simulink model "GridN2"  (R2021a)
settings: Solver=FixedStepAuto  StartTime=0  StopTime=0.2  FixedStep=0.2  RelTol=1e-3
libraries: spsDistributedParametersLineLib x32, spsThreePhaseSeriesRLCLoadLib x10, spsThreePhaseVIMeasurementLib x2, spsGroundLib x1, spsThreePhaseSourceLib x1, spsSeriesRLCBranchLib x1, spspowerguiLib x1
settings Model: Creator=miair  LastModifiedBy=Admin
settings SolverCC: AlgebraicLoopSolver=TrustRegion
settings DebuggingCC: SFMachineParentedDataDiag=warning  ArithmeticOperatorsInVariantConditions=warning
settings SFSimCC: SimUseLocalCustomCode=off  CustomCodeUndefinedFunction=UseInterfaceOnly
settings RTWCC: RTWUseLocalCustomCode=off
settings CodeAppCC: StateflowObjectComments=on
settings SimscapeCC: SimscapeNormalizeSystem=off

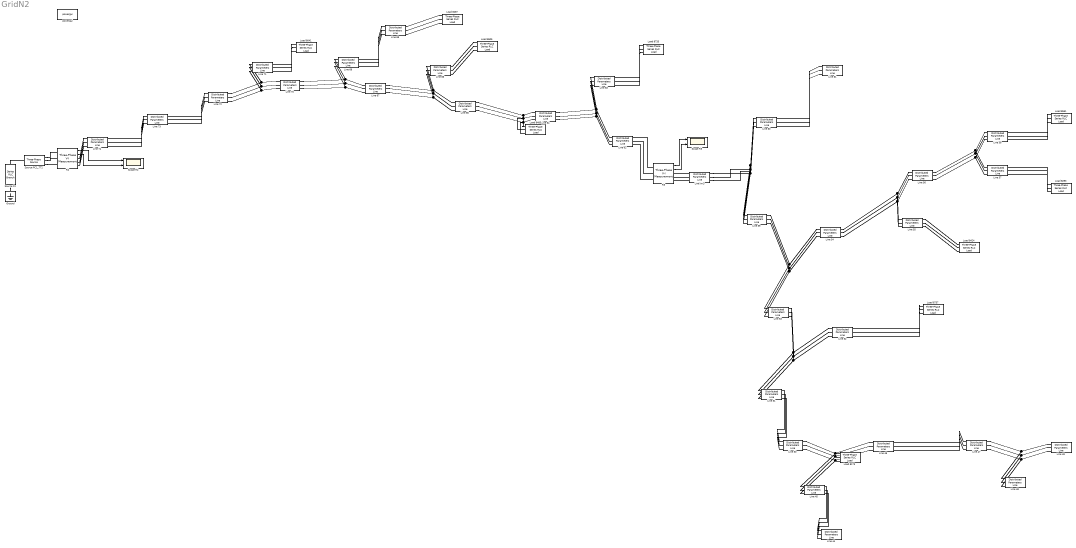
== system GridN2 ==
  Ground : spsGroundLib/Ground  LConnTagsString=a
  Line 44 : spsDistributedParametersLineLib/Distributed Parameters Line  Phases=3  Length=1.11  Frequency=50  Resistance=[0.502970710632245 0.0486237908083191 0.0486712220507153;0.0486237908083191 0.502875844822084 0.0486237934466192;0.0486712220507153 0.0486237934466192 0.502970710632245]  Inductance=[0.00286900545038753 0.00133270803418135 0.00132951476746136;0.00133270803418135 0.00286931445999602 0.00133799988507366;0.00132951476746136 0.00133799988507366 0.00286900545038753]  Capacitance=[8.11484299003193e-09 -1.94249816214699e-09 -1.86930692621136e-09;-1.94249816214699e-09 8.0425699231653e-09 -1.98049571960044e-09;-1.86930692621136e-09 -1.98049571960044e-09 8.13337738722527e-09]  x1=[235.499197131344 9974.6534173124 9973.62003670647;314.159265358979 314.159265358979 314.159265358979;0.999986971190447 -0.174358854278801 -1.7453327880671]  x2=[235.499532901852 9974.66274518172 9973.62938461404;314.159265358979 314.159265358979 314.159265358979;0.999986478978544 -0.1743597320809 -1.74533367343035]  x3=[0.20646047330324 25.3733648317573 25.5655395365313;314.159265358979 314.159265358979 314.159265358979;0.998298068545493 -0.17572688726887 -1.74670236391409]  x4=[0.206460473415381 25.3733648393287 25.5655395441195;314.159265358979 314.159265358979 314.159265358979;0.999986479195967 -0.174359732083028 -1.74533367343085]  x5=5.37516004033389e-06  V1=ones(3,3)  V2=ones(3,3)  I1=ones(3,3)  I2=ones(3,3)  nHarmo=1  Measurements=None  Decoupling=off  VsMag0=0  VrMag0=0  VsAngle0=0  VrAngle0=0  IsMag0=0  IrMag0=0  IsAngle0=0  IrAngle0=0
      settings: SourceProductBaseCode=PS
  Line 45 : spsDistributedParametersLineLib/Distributed Parameters Line  Phases=3  Length=0.03  Frequency=50  Resistance=[0.476003738225748 0.351747138225748 0.351747138225748;0.351747138225748 0.476003738225748 0.351747138225748;0.351747138225748 0.351747138225748 0.476003738225748]  Inductance=[0.000705954362986426 0.000459934243504405 0.000459934243504405;0.000459934243504405 0.000705954362986426 0.000459934243504405;0.000459934243504405 0.000459934243504405 0.000705954362986426]  Capacitance=[5.7561313269996e-07 -1.37543883484145e-07 -1.37543912800485e-07;-1.37543883484145e-07 5.75613027339387e-07 -1.37543875208088e-07;-1.37543912800485e-07 -1.37543875208088e-07 5.75613005057695e-07]  x1=[0.394611268706457 9975.72744348311 9975.73788089302;314.159265358979 314.159265358979 314.159265358979;1.53603881552804 -0.0977008679647626 -1.66848911141861]  x2=[0.394608901343207 9975.72760187554 9975.73803973793;314.159265358979 314.159265358979 314.159265358979;1.53600998571819 -0.0977008934643248 -1.66848913704469]  x3=[0.00519543625612021 537.015102166399 537.015558234621;314.159265358979 314.159265358979 314.159265358979;1.48851023303865 -0.0978903869659834 -1.66867918632059]  x4=[0.0055420607596715 537.015037865136 537.015622619077;314.159265358979 314.159265358979 314.159265358979;1.58036294124239 -0.0976362193465509 -1.66842390704819]  x5=6.63129528657629e-07  V1=ones(3,3)  V2=ones(3,3)  I1=ones(3,3)  I2=ones(3,3)  nHarmo=1  Measurements=None  Decoupling=off  VsMag0=0  VrMag0=0  VsAngle0=0  VrAngle0=0  IsMag0=0  IrMag0=0  IsAngle0=0  IrAngle0=0
      settings: SourceProductBaseCode=PS
  Line 46 : spsDistributedParametersLineLib/Distributed Parameters Line  Phases=3  Length=0.28  Frequency=50  Resistance=[0.476003738225748 0.351747138225748 0.351747138225748;0.351747138225748 0.476003738225748 0.351747138225748;0.351747138225748 0.351747138225748 0.476003738225748]  Inductance=[0.000705954362986426 0.000459934243504405 0.000459934243504405;0.000459934243504405 0.000705954362986426 0.000459934243504405;0.000459934243504405 0.000459934243504405 0.000705954362986426]  Capacitance=[5.7561313269996e-07 -1.37543883484145e-07 -1.37543912800485e-07;-1.37543883484145e-07 5.75613027339387e-07 -1.37543875208088e-07;-1.37543912800485e-07 -1.37543875208088e-07 5.75613005057695e-07]  x1=[0.394611268706457 9975.72744348312 9975.73788089302;314.159265358979 314.159265358979 314.159265358979;1.5343027464817 -0.0987411899313736 -1.6695294333048]  x2=[0.394596540852003 9975.73476310246 9975.7452035338;314.159265358979 314.159265358979 314.159265358979;1.53410803074215 -0.0987423693851286 -1.66953061358232]  x3=[0.0052281315001106 536.342337149453 536.342813729589;314.159265358979 314.159265358979 314.159265358979;1.49901674095737 -0.0999540083208943 -1.67074264139569]  x4=[0.00547168054822011 536.342293969161 536.342857334771;314.159265358979 314.159265358979 314.159265358979;1.56592395108104 -0.0986952571936451 -1.66948311170117]  x5=6.18920893413787e-06  V1=ones(3,3)  V2=ones(3,3)  I1=ones(3,3)  I2=ones(3,3)  nHarmo=1  Measurements=None  Decoupling=off  VsMag0=0  VrMag0=0  VsAngle0=0  VrAngle0=0  IsMag0=0  IrMag0=0  IsAngle0=0  IrAngle0=0
      settings: SourceProductBaseCode=PS
  Line 47 : spsDistributedParametersLineLib/Distributed Parameters Line  Phases=3  Length=0.28  Frequency=50  Resistance=[0.646656091154803 0.0486237908083191 0.0486712220507153;0.0486237908083191 0.646561225344642 0.0486237934466192;0.0486712220507153 0.0486237934466192 0.646656091154803]  Inductance=[0.00282448912315926 0.00133270803418135 0.00132951476746136;0.00133270803418135 0.00282479813276775 0.00133799988507366;0.00132951476746136 0.00133799988507366 0.00282448912315926]  Capacitance=[7.89543174552926e-09 -1.85986777702161e-09 -1.7901190036642e-09;-1.85986777702161e-09 7.82540023894543e-09 -1.8957321828871e-09;-1.7901190036642e-09 -1.8957321828871e-09 7.91264394645417e-09]  x1=[130.165270523337 9974.69985442641 9973.79793227893;314.159265358979 314.159265358979 314.159265358979;1.01815520413661 -0.17955738670952 -1.75050430629446]  x2=[130.1653269492 9974.70262298928 9973.80070570772;314.159265358979 314.159265358979 314.159265358979;1.01815501889747 -0.179557739858097 -1.75050466239578]  x3=[0.113793008832073 25.3764192511602 25.5689515866396;314.159265358979 314.159265358979 314.159265358979;1.01691737955787 -0.180553856209588 -1.75150165648101]  x4=[0.113792232457286 25.3764196987183 25.5689511658165;314.159265358979 314.159265358979 314.159265358979;1.01897135143641 -0.178896144175293 -1.74984250504318]  x5=1.34161235953112e-06  V1=ones(3,3)  V2=ones(3,3)  I1=ones(3,3)  I2=ones(3,3)  nHarmo=1  Measurements=None  Decoupling=off  VsMag0=0  VrMag0=0  VsAngle0=0  VrAngle0=0  IsMag0=0  IrMag0=0  IsAngle0=0  IrAngle0=0
      settings: SourceProductBaseCode=PS
  Line 48 : spsDistributedParametersLineLib/Distributed Parameters Line  Phases=3  Length=0.3  Frequency=50  Resistance=[0.80718830189013 0.0486237908083191 0.0486712220507153;0.0486237908083191 0.807093436079969 0.0486237934466192;0.0486712220507153 0.0486237934466192 0.80718830189013]  Inductance=[0.00279786707424938 0.00133270803418135 0.00132951476746136;0.00133270803418135 0.00279817608385787 0.00133799988507366;0.00132951476746136 0.00133799988507366 0.00279786707424938]  Capacitance=[7.73340098830622e-09 -1.79942827973291e-09 -1.73218055098733e-09;-1.79942827973291e-09 7.66505189233746e-09 -1.83375898618858e-09;-1.73218055098733e-09 -1.83375898618858e-09 7.749673531177e-09]  x1=[52.3203507574151 9974.78925458762 9973.95475226715;314.159265358979 314.159265358979 314.159265358979;1.07773858299054 -0.18388639186805 -1.75479371977811]  x2=[52.3203560131605 9974.78987075889 9973.95536942842;314.159265358979 314.159265358979 314.159265358979;1.07773853006996 -0.183886493366591 -1.75479382212189]  x3=[0.0455873088828184 25.3094904148269 25.5001937895356;314.159265358979 314.159265358979 314.159265358979;1.0772903311148 -0.18423793333454 -1.75514555863699]  x4=[0.0455873088210403 25.3094904150667 25.5001937897322;314.159265358979 314.159265358979 314.159265358979;1.0777385304448 -0.183886493366644 -1.75479382212035]  x5=1.42674452918375e-06  V1=ones(3,3)  V2=ones(3,3)  I1=ones(3,3)  I2=ones(3,3)  nHarmo=1  Measurements=None  Decoupling=off  VsMag0=0  VrMag0=0  VsAngle0=0  VrAngle0=0  IsMag0=0  IrMag0=0  IsAngle0=0  IrAngle0=0
      settings: SourceProductBaseCode=PS
  Line 49 : spsDistributedParametersLineLib/Distributed Parameters Line  Phases=3  Length=0.26  Frequency=50  Resistance=[0.646656091154803 0.0486237908083191 0.0486712220507153;0.0486237908083191 0.646561225344642 0.0486237934466192;0.0486712220507153 0.0486237934466192 0.646656091154803]  Inductance=[0.00282448912315926 0.00133270803418135 0.00132951476746136;0.00133270803418135 0.00282479813276775 0.00133799988507366;0.00132951476746136 0.00133799988507366 0.00282448912315926]  Capacitance=[7.89543174552926e-09 -1.85986777702161e-09 -1.7901190036642e-09;-1.85986777702161e-09 7.82540023894543e-09 -1.8957321828871e-09;-1.7901190036642e-09 -1.8957321828871e-09 7.91264394645417e-09]  x1=[130.165326949199 9974.70262298928 9973.80070570772;314.159265358979 314.159265358979 314.159265358979;1.01818512460841 -0.179533822848032 -1.75048072261842]  x2=[130.16533691815 9974.70310512625 9973.80118871937;314.159265358979 314.159265358979 314.159265358979;1.01818509158021 -0.179533884346449 -1.75048078463717]  x3=[0.113793699489359 25.3769942885345 25.569534921312;314.159265358979 314.159265358979 314.159265358979;1.0177937339126 -0.179844774725389 -1.75079197073384]  x4=[0.113793699536148 25.3769942886748 25.569534921511;314.159265358979 314.159265358979 314.159265358979;1.01818509150153 -0.179533884349861 -1.75048078463657]  x5=1.2457829052789e-06  V1=ones(3,3)  V2=ones(3,3)  I1=ones(3,3)  I2=ones(3,3)  nHarmo=1  Measurements=None  Decoupling=off  VsMag0=0  VrMag0=0  VsAngle0=0  VrAngle0=0  IsMag0=0  IrMag0=0  IsAngle0=0  IrAngle0=0
      settings: SourceProductBaseCode=PS
  Line 50 : spsDistributedParametersLineLib/Distributed Parameters Line  Phases=3  Length=0.02  Frequency=50  Resistance=[0.476003738225748 0.351747138225748 0.351747138225748;0.351747138225748 0.476003738225748 0.351747138225748;0.351747138225748 0.351747138225748 0.476003738225748]  Inductance=[0.000705954362986426 0.000459934243504405 0.000459934243504405;0.000459934243504405 0.000705954362986426 0.000459934243504405;0.000459934243504405 0.000459934243504405 0.000705954362986426]  Capacitance=[5.7561313269996e-07 -1.37543883484145e-07 -1.37543912800485e-07;-1.37543883484145e-07 5.75613027339387e-07 -1.37543875208088e-07;-1.37543912800485e-07 -1.37543875208088e-07 5.75613005057695e-07]  x1=[0.394613836475679 9975.73127591054 9975.74171280773;314.159265358979 314.159265358979 314.159265358979;1.53614175066651 -0.0976590526065954 -1.66844729592049]  x2=[0.394611268706457 9975.72744348312 9975.73788089302;314.159265358979 314.159265358979 314.159265358979;1.5361082582899 -0.0976592550860982 -1.66844749854316]  x3=[0.00508627848822846 535.56585629888 535.566267206896;314.159265358979 314.159265358979 314.159265358979;1.45102711429053 -0.0975036292293395 -1.66829282028614]  x4=[0.00567610136422067 538.518382585317 538.519012218396;314.159265358979 314.159265358979 314.159265358979;1.61223031069708 -0.0978968261558066 -1.66868412697944]  x5=4.42086352438419e-07  V1=ones(3,3)  V2=ones(3,3)  I1=ones(3,3)  I2=ones(3,3)  nHarmo=1  Measurements=None  Decoupling=off  VsMag0=0  VrMag0=0  VsAngle0=0  VrAngle0=0  IsMag0=0  IrMag0=0  IsAngle0=0  IrAngle0=0
      settings: SourceProductBaseCode=PS
  Line 51 : spsDistributedParametersLineLib/Distributed Parameters Line  Phases=3  Length=1.71  Frequency=50  Resistance=[0.646656091154803 0.0486237908083191 0.0486712220507153;0.0486237908083191 0.646561225344642 0.0486237934466192;0.0486712220507153 0.0486237934466192 0.646656091154803]  Inductance=[0.00282448912315926 0.00133270803418135 0.00132951476746136;0.00133270803418135 0.00282479813276775 0.00133799988507366;0.00132951476746136 0.00133799988507366 0.00282448912315926]  Capacitance=[7.89543174552926e-09 -1.85986777702161e-09 -1.7901190036642e-09;-1.85986777702161e-09 7.82540023894543e-09 -1.8957321828871e-09;-1.7901190036642e-09 -1.8957321828871e-09 7.91264394645417e-09]  x1=[130.153869834393 9976.25230830841 9975.34909810887;314.159265358979 314.159265358979 314.159265358979;1.01593395982582 -0.181153028787364 -1.75210222449929]  x2=[130.165195828942 9974.6963681945 9973.79444148245;314.159265358979 314.159265358979 314.159265358979;1.01600469152128 -0.181266070959912 -1.75221461748997]  x3=[0.117758466924286 23.8642665109004 24.0560073748523;314.159265358979 314.159265358979 314.159265358979;0.996810443572246 -0.17982504524178 -1.7508416785956]  x4=[0.109697369932617 26.8098980337402 27.0019891541792;314.159265358979 314.159265358979 314.159265358979;1.03386689924875 -0.184375752260112 -1.75526795592347]  x5=8.19341833856506e-06  V1=ones(3,3)  V2=ones(3,3)  I1=ones(3,3)  I2=ones(3,3)  nHarmo=1  Measurements=None  Decoupling=off  VsMag0=0  VrMag0=0  VsAngle0=0  VrAngle0=0  IsMag0=0  IrMag0=0  IsAngle0=0  IrAngle0=0
      settings: SourceProductBaseCode=PS
  Line 52 : spsDistributedParametersLineLib/Distributed Parameters Line  Phases=3  Length=0.02  Frequency=50  Resistance=[0.646656091154803 0.0486237908083191 0.0486712220507153;0.0486237908083191 0.646561225344642 0.0486237934466192;0.0486712220507153 0.0486237934466192 0.646656091154803]  Inductance=[0.00282448912315926 0.00133270803418135 0.00132951476746136;0.00133270803418135 0.00282479813276775 0.00133799988507366;0.00132951476746136 0.00133799988507366 0.00282448912315926]  Capacitance=[7.89543174552926e-09 -1.85986777702161e-09 -1.7901190036642e-09;-1.85986777702161e-09 7.82540023894543e-09 -1.8957321828871e-09;-1.7901190036642e-09 -1.8957321828871e-09 7.91264394645417e-09]  x1=[130.153869834393 9976.25230830841 9975.34909810887;314.159265358979 314.159265358979 314.159265358979;1.0184778924009 -0.179132041436896 -1.75007931331198]  x2=[130.154016631798 9976.23079318743 9975.32762879486;314.159265358979 314.159265358979 314.159265358979;1.01847831718231 -0.179132357584775 -1.75007962248494]  x3=[0.116739942644273 24.1579696741118 24.3502140022841;314.159265358979 314.159265358979 314.159265358979;0.992668885557271 -0.149703484817279 -1.72089466112461]  x4=[0.110933827863639 26.6377132487628 26.8306479377076;314.159265358979 314.159265358979 314.159265358979;1.04560756980061 -0.205843471298248 -1.77658837325643]  x5=9.5829454252223e-08  V1=ones(3,3)  V2=ones(3,3)  I1=ones(3,3)  I2=ones(3,3)  nHarmo=1  Measurements=None  Decoupling=off  VsMag0=0  VrMag0=0  VsAngle0=0  VrAngle0=0  IsMag0=0  IrMag0=0  IsAngle0=0  IrAngle0=0
      settings: SourceProductBaseCode=PS
  Line 53 : spsDistributedParametersLineLib/Distributed Parameters Line  Phases=3  Length=0.02  Frequency=50  Resistance=[0.646656091154803 0.0486237908083191 0.0486712220507153;0.0486237908083191 0.646561225344642 0.0486237934466192;0.0486712220507153 0.0486237934466192 0.646656091154803]  Inductance=[0.00282448912315926 0.00133270803418135 0.00132951476746136;0.00133270803418135 0.00282479813276775 0.00133799988507366;0.00132951476746136 0.00133799988507366 0.00282448912315926]  Capacitance=[7.89543174552926e-09 -1.85986777702161e-09 -1.7901190036642e-09;-1.85986777702161e-09 7.82540023894543e-09 -1.8957321828871e-09;-1.7901190036642e-09 -1.8957321828871e-09 7.91264394645417e-09]  x1=[130.153585411917 9976.29177268076 9975.38850120097;314.159265358979 314.159265358979 314.159265358979;1.01847665737296 -0.179130371531821 -1.75007765770378]  x2=[130.153869834393 9976.25230830841 9975.34909810887;314.159265358979 314.159265358979 314.159265358979;1.0184778924009 -0.179132041436896 -1.75007931331198]  x3=[0.120851509252682 22.6831177191226 22.8750937750787;314.159265358979 314.159265358979 314.159265358979;0.974863217260378 -0.146414702078281 -1.71770900196937]  x4=[0.106986770746654 28.1147049917407 28.3078095934207;314.159265358979 314.159265358979 314.159265358979;1.06771566347072 -0.205547045337112 -1.77625580935564]  x5=9.5829454252223e-08  V1=ones(3,3)  V2=ones(3,3)  I1=ones(3,3)  I2=ones(3,3)  nHarmo=1  Measurements=None  Decoupling=off  VsMag0=0  VrMag0=0  VsAngle0=0  VrAngle0=0  IsMag0=0  IrMag0=0  IsAngle0=0  IrAngle0=0
      settings: SourceProductBaseCode=PS
  Line 54 : spsDistributedParametersLineLib/Distributed Parameters Line  Phases=3  Length=1.15  Frequency=50  Resistance=[0.646656091154803 0.0486237908083191 0.0486712220507153;0.0486237908083191 0.646561225344642 0.0486237934466192;0.0486712220507153 0.0486237934466192 0.646656091154803]  Inductance=[0.00282448912315926 0.00133270803418135 0.00132951476746136;0.00133270803418135 0.00282479813276775 0.00133799988507366;0.00132951476746136 0.00133799988507366 0.00282448912315926]  Capacitance=[7.89543174552926e-09 -1.85986777702161e-09 -1.7901190036642e-09;-1.85986777702161e-09 7.82540023894543e-09 -1.8957321828871e-09;-1.7901190036642e-09 -1.8957321828871e-09 7.91264394645417e-09]  x1=[130.153585411917 9976.29177268076 9975.38850120097;314.159265358979 314.159265358979 314.159265358979;1.01677568470442 -0.180481682600477 -1.75143025512488]  x2=[130.16626652108 9974.54734273492 9973.6476594975;314.159265358979 314.159265358979 314.159265358979;1.01681332557288 -0.180520999955708 -1.75146901015184]  x3=[0.118237518025689 23.5272003979984 23.7187520710131;314.159265358979 314.159265358979 314.159265358979;0.977882363618498 -0.143839943823494 -1.71513126174304]  x4=[0.109419951312209 27.2095212764847 27.4020023602839;314.159265358979 314.159265358979 314.159265358979;1.0570428697276 -0.21348210988213 -1.78416900813399]  x5=5.51019361950282e-06  V1=ones(3,3)  V2=ones(3,3)  I1=ones(3,3)  I2=ones(3,3)  nHarmo=1  Measurements=None  Decoupling=off  VsMag0=0  VrMag0=0  VsAngle0=0  VrAngle0=0  IsMag0=0  IrMag0=0  IsAngle0=0  IrAngle0=0
      settings: SourceProductBaseCode=PS
  Line 55 : spsDistributedParametersLineLib/Distributed Parameters Line  Phases=3  Length=0.19  Frequency=50  Resistance=[0.646656091154803 0.0486237908083191 0.0486712220507153;0.0486237908083191 0.646561225344642 0.0486237934466192;0.0486712220507153 0.0486237934466192 0.646656091154803]  Inductance=[0.00282448912315926 0.00133270803418135 0.00132951476746136;0.00133270803418135 0.00282479813276775 0.00133799988507366;0.00132951476746136 0.00133799988507366 0.00282448912315926]  Capacitance=[7.89543174552926e-09 -1.85986777702161e-09 -1.7901190036642e-09;-1.85986777702161e-09 7.82540023894543e-09 -1.8957321828871e-09;-1.7901190036642e-09 -1.8957321828871e-09 7.91264394645417e-09]  x1=[130.16626652108 9974.54734273492 9973.6476594975;314.159265358979 314.159265358979 314.159265358979;1.01825839969837 -0.179372983472602 -1.75031990083834]  x2=[130.167047937169 9974.43157979928 9973.53211570487;314.159265358979 314.159265358979 314.159265358979;1.01826120436805 -0.179375704015156 -1.75032258160693]  x3=[0.115619383091202 24.6351358497311 24.8275074767809;314.159265358979 314.159265358979 314.159265358979;1.00420677217725 -0.165387593021386 -1.73645187255032]  x4=[0.112000815304933 26.1265781592648 26.3193115756065;314.159265358979 314.159265358979 314.159265358979;1.03247625999877 -0.192783350721144 -1.76362543182429]  x5=9.10379815396118e-07  V1=ones(3,3)  V2=ones(3,3)  I1=ones(3,3)  I2=ones(3,3)  nHarmo=1  Measurements=None  Decoupling=off  VsMag0=0  VrMag0=0  VsAngle0=0  VrAngle0=0  IsMag0=0  IrMag0=0  IsAngle0=0  IrAngle0=0
      settings: SourceProductBaseCode=PS
  Line 56 : spsDistributedParametersLineLib/Distributed Parameters Line  Phases=3  Length=0.34  Frequency=50  Resistance=[0.646656091154803 0.0486237908083191 0.0486712220507153;0.0486237908083191 0.646561225344642 0.0486237934466192;0.0486712220507153 0.0486237934466192 0.646656091154803]  Inductance=[0.00282448912315926 0.00133270803418135 0.00132951476746136;0.00133270803418135 0.00282479813276775 0.00133799988507366;0.00132951476746136 0.00133799988507366 0.00282448912315926]  Capacitance=[7.89543174552926e-09 -1.85986777702161e-09 -1.7901190036642e-09;-1.85986777702161e-09 7.82540023894543e-09 -1.8957321828871e-09;-1.7901190036642e-09 -1.8957321828871e-09 7.91264394645417e-09]  x1=[130.16626652108 9974.54734273492 9973.6476594975;314.159265358979 314.159265358979 314.159265358979;1.01803260686626 -0.179552361048087 -1.75049944916857]  x2=[130.168533192606 9974.23468143005 9973.33565944929;314.159265358979 314.159265358979 314.159265358979;1.01803899443892 -0.179558599592712 -1.7505055881998]  x3=[0.116428678428167 24.2813500041598 24.4735087715179;314.159265358979 314.159265358979 314.159265358979;0.994175597165718 -0.156785395571565 -1.72793500970604]  x4=[0.111219856893532 26.4787015727691 26.6714385911402;314.159265358979 314.159265358979 314.159265358979;1.04248987173781 -0.200825449479797 -1.77160026552266]  x5=1.62910072228779e-06  V1=ones(3,3)  V2=ones(3,3)  I1=ones(3,3)  I2=ones(3,3)  nHarmo=1  Measurements=None  Decoupling=off  VsMag0=0  VrMag0=0  VsAngle0=0  VrAngle0=0  IsMag0=0  IrMag0=0  IsAngle0=0  IrAngle0=0
      settings: SourceProductBaseCode=PS
  Line 57 : spsDistributedParametersLineLib/Distributed Parameters Line  Phases=3  Length=0.12  Frequency=50  Resistance=[0.646656091154803 0.0486237908083191 0.0486712220507153;0.0486237908083191 0.646561225344642 0.0486237934466192;0.0486712220507153 0.0486237934466192 0.646656091154803]  Inductance=[0.00282448912315926 0.00133270803418135 0.00132951476746136;0.00133270803418135 0.00282479813276775 0.00133799988507366;0.00132951476746136 0.00133799988507366 0.00282448912315926]  Capacitance=[7.89543174552926e-09 -1.85986777702161e-09 -1.7901190036642e-09;-1.85986777702161e-09 7.82540023894543e-09 -1.8957321828871e-09;-1.7901190036642e-09 -1.8957321828871e-09 7.91264394645417e-09]  x1=[130.168533192606 9974.23468143005 9973.33565944929;314.159265358979 314.159265358979 314.159265358979;1.01837015725935 -0.179295512482 -1.75024225064879]  x2=[130.168728242859 9974.20541837634 9973.30644537064;314.159265358979 314.159265358979 314.159265358979;1.01837098801547 -0.179296434605923 -1.75024316218331]  x3=[0.114590526949465 25.0657437692469 25.2582728779101;314.159265358979 314.159265358979 314.159265358979;1.01299458112372 -0.174624175193014 -1.74561076889279]  x4=[0.113021369127735 25.6944524930637 25.8871185087763;314.159265358979 314.159265358979 314.159265358979;1.02363931189864 -0.183995211306265 -1.75490402542678]  x5=5.74976725513338e-07  V1=ones(3,3)  V2=ones(3,3)  I1=ones(3,3)  I2=ones(3,3)  nHarmo=1  Measurements=None  Decoupling=off  VsMag0=0  VrMag0=0  VsAngle0=0  VrAngle0=0  IsMag0=0  IrMag0=0  IsAngle0=0  IrAngle0=0
      settings: SourceProductBaseCode=PS
  Line 58 : spsDistributedParametersLineLib/Distributed Parameters Line  Phases=3  Length=0.82  Frequency=50  Resistance=[0.646656091154803 0.0486237908083191 0.0486712220507153;0.0486237908083191 0.646561225344642 0.0486237934466192;0.0486712220507153 0.0486237934466192 0.646656091154803]  Inductance=[0.00282448912315926 0.00133270803418135 0.00132951476746136;0.00133270803418135 0.00282479813276775 0.00133799988507366;0.00132951476746136 0.00133799988507366 0.00282448912315926]  Capacitance=[7.89543174552926e-09 -1.85986777702161e-09 -1.7901190036642e-09;-1.85986777702161e-09 7.82540023894543e-09 -1.8957321828871e-09;-1.7901190036642e-09 -1.8957321828871e-09 7.91264394645417e-09]  x1=[130.168533192606 9974.23468143005 9973.3356594493;314.159265358979 314.159265358979 314.159265358979;1.01731645737618 -0.180132607834265 -1.75108014285655]  x2=[130.172512252034 9973.67309540897 9972.77531994938;314.159265358979 314.159265358979 314.159265358979;1.01732669809245 -0.180140398631069 -1.75108775791298]  x3=[0.115605201111395 24.5790296267231 24.7710683323559;314.159265358979 314.159265358979 314.159265358979;0.99912525799645 -0.161992460376518 -1.73309623231583]  x4=[0.111965570108671 26.1470133803964 26.3394813325676;314.159265358979 314.159265358979 314.159265358979;1.0348548985309 -0.198143858065956 -1.76895306273468]  x5=3.92900762434114e-06  V1=ones(3,3)  V2=ones(3,3)  I1=ones(3,3)  I2=ones(3,3)  nHarmo=1  Measurements=None  Decoupling=off  VsMag0=0  VrMag0=0  VsAngle0=0  VrAngle0=0  IsMag0=0  IrMag0=0  IsAngle0=0  IrAngle0=0
      settings: SourceProductBaseCode=PS
  Line 59 : spsDistributedParametersLineLib/Distributed Parameters Line  Phases=3  Length=1.11  Frequency=50  Resistance=[0.646656091154803 0.0486237908083191 0.0486712220507153;0.0486237908083191 0.646561225344642 0.0486237934466192;0.0486712220507153 0.0486237934466192 0.646656091154803]  Inductance=[0.00282448912315926 0.00133270803418135 0.00132951476746136;0.00133270803418135 0.00282479813276775 0.00133799988507366;0.00132951476746136 0.00133799988507366 0.00282448912315926]  Capacitance=[7.89543174552926e-09 -1.85986777702161e-09 -1.7901190036642e-09;-1.85986777702161e-09 7.82540023894543e-09 -1.8957321828871e-09;-1.7901190036642e-09 -1.8957321828871e-09 7.91264394645417e-09]  x1=[130.125187558168 9980.14784167935 9979.23767099196;314.159265358979 314.159265358979 314.159265358979;1.01673223065322 -0.18030097498308 -1.75125081803133]  x2=[130.153585411918 9976.29177268076 9975.38850120097;314.159265358979 314.159265358979 314.159265358979;1.01683589612632 -0.180433848580348 -1.75138237557016]  x3=[0.125467447253769 20.8669248157678 21.0574267772761;314.159265358979 314.159265358979 314.159265358979;0.936516761246663 -0.104982283798124 -1.67676040712555]  x4=[0.102859050266621 29.9580417153643 30.1507990404979;314.159265358979 314.159265358979 314.159265358979;1.11288919169921 -0.23397617246079 -1.80449026431088]  x5=5.31853471099837e-06  V1=ones(3,3)  V2=ones(3,3)  I1=ones(3,3)  I2=ones(3,3)  nHarmo=1  Measurements=None  Decoupling=off  VsMag0=0  VrMag0=0  VsAngle0=0  VrAngle0=0  IsMag0=0  IrMag0=0  IsAngle0=0  IrAngle0=0
      settings: SourceProductBaseCode=PS
  Line 60 : spsDistributedParametersLineLib/Distributed Parameters Line  Phases=3  Length=0.21  Frequency=50  Resistance=[0.646656091154803 0.0486237908083191 0.0486712220507153;0.0486237908083191 0.646561225344642 0.0486237934466192;0.0486712220507153 0.0486237934466192 0.646656091154803]  Inductance=[0.00282448912315926 0.00133270803418135 0.00132951476746136;0.00133270803418135 0.00282479813276775 0.00133799988507366;0.00132951476746136 0.00133799988507366 0.00282448912315926]  Capacitance=[7.89543174552926e-09 -1.85986777702161e-09 -1.7901190036642e-09;-1.85986777702161e-09 7.82540023894543e-09 -1.8957321828871e-09;-1.7901190036642e-09 -1.8957321828871e-09 7.91264394645417e-09]  x1=[130.125187558168 9980.14784167935 9979.23767099195;314.159265358979 314.159265358979 314.159265358979;1.01808698764586 -0.179224709530169 -1.75017352804992]  x2=[130.124739331175 9980.19890685876 9979.28842161734;314.159265358979 314.159265358979 314.159265358979;1.01808986437633 -0.179231221533039 -1.75018003909566]  x3=[0.11419217761102 25.3975537040212 25.5903096333728;314.159265358979 314.159265358979 314.159265358979;1.03038026904643 -0.199727722033007 -1.77052636969296]  x4=[0.113347937314895 25.3977092018999 25.590172958523;314.159265358979 314.159265358979 314.159265358979;1.00538772769245 -0.158979482471346 -1.73007847733232]  x5=1.00620926964834e-06  V1=ones(3,3)  V2=ones(3,3)  I1=ones(3,3)  I2=ones(3,3)  nHarmo=1  Measurements=None  Decoupling=off  VsMag0=0  VrMag0=0  VsAngle0=0  VrAngle0=0  IsMag0=0  IrMag0=0  IsAngle0=0  IrAngle0=0
      settings: SourceProductBaseCode=PS
  Line 61 : spsDistributedParametersLineLib/Distributed Parameters Line  Phases=3  Length=0.23  Frequency=50  Resistance=[0.476003738225748 0.351747138225748 0.351747138225748;0.351747138225748 0.476003738225748 0.351747138225748;0.351747138225748 0.351747138225748 0.476003738225748]  Inductance=[0.000705954362986426 0.000459934243504405 0.000459934243504405;0.000459934243504405 0.000705954362986426 0.000459934243504405;0.000459934243504405 0.000459934243504405 0.000705954362986426]  Capacitance=[5.7561313269996e-07 -1.37543883484145e-07 -1.37543912800485e-07;-1.37543883484145e-07 5.75613027339387e-07 -1.37543875208088e-07;-1.37543912800485e-07 -1.37543875208088e-07 5.75613005057695e-07]  x1=[0.270768221935307 9981.23593924016 9981.23548031225;314.159265358979 314.159265358979 314.159265358979;1.56817561453902 -0.0982919037173954 -1.66908199249218]  x2=[0.270768567313193 9981.24051081139 9981.24005188258;314.159265358979 314.159265358979 314.159265358979;1.56817266915462 -0.0982926400606238 -1.6690827288353]  x3=[0.0036711401576612 536.772956923946 536.772890796409;314.159265358979 314.159265358979 314.159265358979;1.56657697956209 -0.0992493680983301 -1.6700394567994]  x4=[0.00367114003873441 536.772957018554 536.772890890006;314.159265358979 314.159265358979 314.159265358979;1.56817266008994 -0.0982926400608598 -1.66908272883497]  x5=5.08399305304182e-06  V1=ones(3,3)  V2=ones(3,3)  I1=ones(3,3)  I2=ones(3,3)  nHarmo=1  Measurements=None  Decoupling=off  VsMag0=0  VrMag0=0  VsAngle0=0  VrAngle0=0  IsMag0=0  IrMag0=0  IsAngle0=0  IrAngle0=0
      settings: SourceProductBaseCode=PS
  Line 62 : spsDistributedParametersLineLib/Distributed Parameters Line  Phases=3  Length=0.24  Frequency=50  Resistance=[0.646656091154803 0.0486237908083191 0.0486712220507153;0.0486237908083191 0.646561225344642 0.0486237934466192;0.0486712220507153 0.0486237934466192 0.646656091154803]  Inductance=[0.00282448912315926 0.00133270803418135 0.00132951476746136;0.00133270803418135 0.00282479813276775 0.00133799988507366;0.00132951476746136 0.00133799988507366 0.00282448912315926]  Capacitance=[7.89543174552926e-09 -1.85986777702161e-09 -1.7901190036642e-09;-1.85986777702161e-09 7.82540023894543e-09 -1.8957321828871e-09;-1.7901190036642e-09 -1.8957321828871e-09 7.91264394645417e-09]  x1=[130.122951158228 9980.92057997789 9980.01126648648;314.159265358979 314.159265358979 314.159265358979;1.01799768682142 -0.179224187935843 -1.7501734823709]  x2=[130.125187558175 9980.14784167968 9979.23767099227;314.159265358979 314.159265358979 314.159265358979;1.0180418290795 -0.17926058504525 -1.75020943771595]  x3=[0.127447172807473 20.8616193035841 21.0504212049552;314.159265358979 314.159265358979 314.159265358979;1.02169241408167 -0.128978012605352 -1.69988289206204]  x4=[0.100072442182212 29.9681379680079 30.1651549342218;314.159265358979 314.159265358979 314.159265358979;1.01293174588384 -0.214468512605215 -1.78553497084211]  x5=1.14995345102668e-06  V1=ones(3,3)  V2=ones(3,3)  I1=ones(3,3)  I2=ones(3,3)  nHarmo=1  Measurements=None  Decoupling=off  VsMag0=0  VrMag0=0  VsAngle0=0  VrAngle0=0  IsMag0=0  IrMag0=0  IsAngle0=0  IrAngle0=0
      settings: SourceProductBaseCode=PS
  Line 63 : spsDistributedParametersLineLib/Distributed Parameters Line  Phases=3  Length=0.02  Frequency=50  Resistance=[0.646656091154803 0.0486237908083191 0.0486712220507153;0.0486237908083191 0.646561225344642 0.0486237934466192;0.0486712220507153 0.0486237934466192 0.646656091154803]  Inductance=[0.00282448912315926 0.00133270803418135 0.00132951476746136;0.00133270803418135 0.00282479813276775 0.00133799988507366;0.00132951476746136 0.00133799988507366 0.00282448912315926]  Capacitance=[7.89543174552926e-09 -1.85986777702161e-09 -1.7901190036642e-09;-1.85986777702161e-09 7.82540023894543e-09 -1.8957321828871e-09;-1.7901190036642e-09 -1.8957321828871e-09 7.91264394645417e-09]  x1=[130.122951158228 9980.92057997789 9980.01126648648;314.159265358979 314.159265358979 314.159265358979;1.01832884964184 -0.178961100825132 -1.74991014481989]  x2=[130.122998810064 9980.9137618374 9980.00446489494;314.159265358979 314.159265358979 314.159265358979;1.01832894624436 -0.178961130799039 -1.74991017275917]  x3=[0.114585658231989 25.0365098210977 25.2291329828466;314.159265358979 314.159265358979 314.159265358979;1.0092887177429 -0.168525816343045 -1.7395577200327]  x4=[0.112963659285141 25.7657017891028 25.9585535894843;314.159265358979 314.159265358979 314.159265358979;1.02746856385999 -0.189124655596812 -1.75999529351849]  x5=9.5829454252223e-08  V1=ones(3,3)  V2=ones(3,3)  I1=ones(3,3)  I2=ones(3,3)  nHarmo=1  Measurements=None  Decoupling=off  VsMag0=0  VrMag0=0  VsAngle0=0  VrAngle0=0  IsMag0=0  IrMag0=0  IsAngle0=0  IrAngle0=0
      settings: SourceProductBaseCode=PS
  Line 64 : spsDistributedParametersLineLib/Distributed Parameters Line  Phases=3  Length=0.5  Frequency=50  Resistance=[0.646656091154803 0.0486237908083191 0.0486712220507153;0.0486237908083191 0.646561225344642 0.0486237934466192;0.0486712220507153 0.0486237934466192 0.646656091154803]  Inductance=[0.00282448912315926 0.00133270803418135 0.00132951476746136;0.00133270803418135 0.00282479813276775 0.00133799988507366;0.00132951476746136 0.00133799988507366 0.00282448912315926]  Capacitance=[7.89543174552926e-09 -1.85986777702161e-09 -1.7901190036642e-09;-1.85986777702161e-09 7.82540023894543e-09 -1.8957321828871e-09;-1.7901190036642e-09 -1.8957321828871e-09 7.91264394645417e-09]  x1=[130.117045517735 9982.69823616629 9981.79028878362;314.159265358979 314.159265358979 314.159265358979;1.01751211428612 -0.179458206265749 -1.75040876473354]  x2=[130.122951158228 9980.92057997788 9980.01126648648;314.159265358979 314.159265358979 314.159265358979;1.0176063125791 -0.179535109066685 -1.75048469947664]  x3=[0.128238198810166 20.5096498041529 20.6982529021976;314.159265358979 314.159265358979 314.159265358979;1.01245042115513 -0.116327600818977 -1.6873605130524]  x4=[0.0992466536391 30.3357905879267 30.5328316950016;314.159265358979 314.159265358979 314.159265358979;1.0232977416096 -0.222689996530779 -1.79369961338263]  x5=2.39573635630557e-06  V1=ones(3,3)  V2=ones(3,3)  I1=ones(3,3)  I2=ones(3,3)  nHarmo=1  Measurements=None  Decoupling=off  VsMag0=0  VrMag0=0  VsAngle0=0  VrAngle0=0  IsMag0=0  IrMag0=0  IsAngle0=0  IrAngle0=0
      settings: SourceProductBaseCode=PS
  Line 65 : spsDistributedParametersLineLib/Distributed Parameters Line  Phases=3  Length=0.23  Frequency=50  Resistance=[0.646656091154803 0.0486237908083191 0.0486712220507153;0.0486237908083191 0.646561225344642 0.0486237934466192;0.0486712220507153 0.0486237934466192 0.646656091154803]  Inductance=[0.00282448912315926 0.00133270803418135 0.00132951476746136;0.00133270803418135 0.00282479813276775 0.00133799988507366;0.00132951476746136 0.00133799988507366 0.00282448912315926]  Capacitance=[7.89543174552926e-09 -1.85986777702161e-09 -1.7901190036642e-09;-1.85986777702161e-09 7.82540023894543e-09 -1.8957321828871e-09;-1.7901190036642e-09 -1.8957321828871e-09 7.91264394645417e-09]  x1=[130.11129265089 9983.97610165688 9983.06804616825;314.159265358979 314.159265358979 314.159265358979;1.0178614846406 -0.179084390056721 -1.75003525581554]  x2=[130.117045517735 9982.69823616629 9981.79028878362;314.159265358979 314.159265358979 314.159265358979;1.01791854138391 -0.179135326629876 -1.75008557773912]  x3=[0.134948050658406 17.9998369016738 18.1874946490578;314.159265358979 314.159265358979 314.159265358979;0.977454089984401 -0.0551384442101795 -1.62684864252585]  x4=[0.0928216512913186 33.0135527681553 33.2112399363187;314.159265358979 314.159265358979 314.159265358979;1.07627031656615 -0.246792546271566 -1.81762794115397]  x5=1.10203872390056e-06  V1=ones(3,3)  V2=ones(3,3)  I1=ones(3,3)  I2=ones(3,3)  nHarmo=1  Measurements=None  Decoupling=off  VsMag0=0  VrMag0=0  VsAngle0=0  VrAngle0=0  IsMag0=0  IrMag0=0  IsAngle0=0  IrAngle0=0
      settings: SourceProductBaseCode=PS
  Line 66 : spsDistributedParametersLineLib/Distributed Parameters Line  Phases=3  Length=1.62  Frequency=50  Resistance=[0.80718830189013 0.0486237908083191 0.0486712220507153;0.0486237908083191 0.807093436079969 0.0486237934466192;0.0486712220507153 0.0486237934466192 0.80718830189013]  Inductance=[0.00279786707424938 0.00133270803418135 0.00132951476746136;0.00133270803418135 0.00279817608385787 0.00133799988507366;0.00132951476746136 0.00133799988507366 0.00279786707424938]  Capacitance=[7.73340098830622e-09 -1.79942827973291e-09 -1.73218055098733e-09;-1.79942827973291e-09 7.66505189233746e-09 -1.83375898618858e-09;-1.73218055098733e-09 -1.83375898618858e-09 7.749673531177e-09]  x1=[52.1881099981272 9984.0626797127 9983.22183237434;314.159265358979 314.159265358979 314.159265358979;1.07443756256919 -0.185019415932358 -1.75593203967872]  x2=[52.1886317469232 9984.04958880798 9983.20881654872;314.159265358979 314.159265358979 314.159265358979;1.07443943521712 -0.185022758290388 -1.75593539758709]  x3=[0.0455419917273008 25.2650140138692 25.4551508418951;314.159265358979 314.159265358979 314.159265358979;1.07032147367503 -0.186566187363917 -1.75748319798191]  x4=[0.0453322417537417 25.3045666845579 25.4947105245434;314.159265358979 314.159265358979 314.159265358979;1.07614778540612 -0.18537644712688 -1.75628631426717]  x5=7.70442045759223e-06  V1=ones(3,3)  V2=ones(3,3)  I1=ones(3,3)  I2=ones(3,3)  nHarmo=1  Measurements=None  Decoupling=off  VsMag0=0  VrMag0=0  VsAngle0=0  VrAngle0=0  IsMag0=0  IrMag0=0  IsAngle0=0  IrAngle0=0
      settings: SourceProductBaseCode=PS
  Line 67 : spsDistributedParametersLineLib/Distributed Parameters Line  Phases=3  Length=0.54  Frequency=50  Resistance=[0.646656091154803 0.0486237908083191 0.0486712220507153;0.0486237908083191 0.646561225344642 0.0486237934466192;0.0486712220507153 0.0486237934466192 0.646656091154803]  Inductance=[0.00282448912315926 0.00133270803418135 0.00132951476746136;0.00133270803418135 0.00282479813276775 0.00133799988507366;0.00132951476746136 0.00133799988507366 0.00282448912315926]  Capacitance=[7.89543174552926e-09 -1.85986777702161e-09 -1.7901190036642e-09;-1.85986777702161e-09 7.82540023894543e-09 -1.8957321828871e-09;-1.7901190036642e-09 -1.8957321828871e-09 7.91264394645417e-09]  x1=[130.097424952485 9986.96991682868 9986.06156319385;314.159265358979 314.159265358979 314.159265358979;1.01726164043262 -0.179333417153171 -1.75028606531289]  x2=[130.111292650889 9983.97610165688 9983.06804616825;314.159265358979 314.159265358979 314.159265358979;1.01739484612091 -0.179455103712724 -1.7504063223647]  x3=[0.134984287429377 17.9740865519816 18.1616480714255;314.159265358979 314.159265358979 314.159265358979;0.973963233484223 -0.0582994610414948 -1.63001273218046]  x4=[0.0927713304025912 33.0226386664014 33.2201771766931;314.159265358979 314.159265358979 314.159265358979;1.07944891402359 -0.245689959058695 -1.81652075252842]  x5=2.58739526481002e-06  V1=ones(3,3)  V2=ones(3,3)  I1=ones(3,3)  I2=ones(3,3)  nHarmo=1  Measurements=None  Decoupling=off  VsMag0=0  VrMag0=0  VsAngle0=0  VrAngle0=0  IsMag0=0  IrMag0=0  IsAngle0=0  IrAngle0=0
      settings: SourceProductBaseCode=PS
  Line 68 : spsDistributedParametersLineLib/Distributed Parameters Line  Phases=3  Length=0.14  Frequency=50  Resistance=[0.646656091154803 0.0486237908083191 0.0486712220507153;0.0486237908083191 0.646561225344642 0.0486237934466192;0.0486712220507153 0.0486237934466192 0.646656091154803]  Inductance=[0.00282448912315926 0.00133270803418135 0.00132951476746136;0.00133270803418135 0.00282479813276775 0.00133799988507366;0.00132951476746136 0.00133799988507366 0.00282448912315926]  Capacitance=[7.89543174552926e-09 -1.85986777702161e-09 -1.7901190036642e-09;-1.85986777702161e-09 7.82540023894543e-09 -1.8957321828871e-09;-1.7901190036642e-09 -1.8957321828871e-09 7.91264394645417e-09]  x1=[130.097424952485 9986.96991682868 9986.06156319385;314.159265358979 314.159265358979 314.159265358979;1.01786375465157 -0.178855076951876 -1.74980726976559]  x2=[130.099322577909 9986.69325396292 9985.78550327928;314.159265358979 314.159265358979 314.159265358979;1.01786897386625 -0.178858684825675 -1.7498107892724]  x3=[0.119111876769318 23.1981757660137 23.3900194592326;314.159265358979 314.159265358979 314.159265358979;0.970615264483877 -0.121166352551498 -1.69261496666521]  x4=[0.108649196578431 27.6956021369787 27.8887905632008;314.159265358979 314.159265358979 314.159265358979;1.06945061933574 -0.227324967675718 -1.79792332886751]  x5=6.70806179765561e-07  V1=ones(3,3)  V2=ones(3,3)  I1=ones(3,3)  I2=ones(3,3)  nHarmo=1  Measurements=None  Decoupling=off  VsMag0=0  VrMag0=0  VsAngle0=0  VrAngle0=0  IsMag0=0  IrMag0=0  IsAngle0=0  IrAngle0=0
      settings: SourceProductBaseCode=PS
  Line 69 : spsDistributedParametersLineLib/Distributed Parameters Line  Phases=3  Length=0.15  Frequency=50  Resistance=[0.476003738225748 0.351747138225748 0.351747138225748;0.351747138225748 0.476003738225748 0.351747138225748;0.351747138225748 0.351747138225748 0.476003738225748]  Inductance=[0.000705954362986426 0.000459934243504405 0.000459934243504405;0.000459934243504405 0.000705954362986426 0.000459934243504405;0.000459934243504405 0.000459934243504405 0.000705954362986426]  Capacitance=[5.7561313269996e-07 -1.37543883484145e-07 -1.37543912800485e-07;-1.37543883484145e-07 5.75613027339387e-07 -1.37543875208088e-07;-1.37543912800485e-07 -1.37543875208088e-07 5.75613005057695e-07]  x1=[0.135487675673386 9987.7336710225 9987.73135937569;314.159265358979 314.159265358979 314.159265358979;1.49453808066144 -0.0976701424658557 -1.6684636285827]  x2=[0.13548775677929 9987.67419429578 9987.67188266243;314.159265358979 314.159265358979 314.159265358979;1.49453690917889 -0.0976699403464067 -1.6684634264632]  x3=[0.00183879953689306 535.088293628895 535.088128275934;314.159265358979 314.159265358979 314.159265358979;1.49351577983918 -0.0951644528310238 -1.66595793865545]  x4=[0.00183868203158694 539.588327542272 539.588161147428;314.159265358979 314.159265358979 314.159265358979;1.49451692082746 -0.100776480241083 -1.67156996659784]  x5=3.31564764328815e-06  V1=ones(3,3)  V2=ones(3,3)  I1=ones(3,3)  I2=ones(3,3)  nHarmo=1  Measurements=None  Decoupling=off  VsMag0=0  VrMag0=0  VsAngle0=0  VrAngle0=0  IsMag0=0  IrMag0=0  IsAngle0=0  IrAngle0=0
      settings: SourceProductBaseCode=PS
  Line 70 : spsDistributedParametersLineLib/Distributed Parameters Line  Phases=3  Length=0.5  Frequency=50  Resistance=[0.646656091154803 0.0486237908083191 0.0486712220507153;0.0486237908083191 0.646561225344642 0.0486237934466192;0.0486712220507153 0.0486237934466192 0.646656091154803]  Inductance=[0.00282448912315926 0.00133270803418135 0.00132951476746136;0.00133270803418135 0.00282479813276775 0.00133799988507366;0.00132951476746136 0.00133799988507366 0.00282448912315926]  Capacitance=[7.89543174552926e-09 -1.85986777702161e-09 -1.7901190036642e-09;-1.85986777702161e-09 7.82540023894543e-09 -1.8957321828871e-09;-1.7901190036642e-09 -1.8957321828871e-09 7.91264394645417e-09]  x1=[130.077722677422 9990.72598437802 9989.81518997748;314.159265358979 314.159265358979 314.159265358979;1.01718012658065 -0.179159569904418 -1.75011380615577]  x2=[130.097424952485 9986.96991682868 9986.06156319385;314.159265358979 314.159265358979 314.159265358979;1.01732185185452 -0.179285583133041 -1.75023818575816]  x3=[0.140557372228566 15.9883610781046 16.1729817061025;314.159265358979 314.159265358979 314.159265358979;0.934915850041807 0.041116425819239 -1.53187035624163]  x4=[0.0880940851986396 35.3847071749531 35.5826356356809;314.159265358979 314.159265358979 314.159265358979;1.14787090583191 -0.278570478838234 -1.84920621049723]  x5=2.39573635630557e-06  V1=ones(3,3)  V2=ones(3,3)  I1=ones(3,3)  I2=ones(3,3)  nHarmo=1  Measurements=None  Decoupling=off  VsMag0=0  VrMag0=0  VsAngle0=0  VrAngle0=0  IsMag0=0  IrMag0=0  IsAngle0=0  IrAngle0=0
      settings: SourceProductBaseCode=PS
  Line 71 : spsDistributedParametersLineLib/Distributed Parameters Line  Phases=3  Length=0.17  Frequency=50  Resistance=[0.646656091154803 0.0486237908083191 0.0486712220507153;0.0486237908083191 0.646561225344642 0.0486237934466192;0.0486712220507153 0.0486237934466192 0.646656091154803]  Inductance=[0.00282448912315926 0.00133270803418135 0.00132951476746136;0.00133270803418135 0.00282479813276775 0.00133799988507366;0.00132951476746136 0.00133799988507366 0.00282448912315926]  Capacitance=[7.89543174552926e-09 -1.85986777702161e-09 -1.7901190036642e-09;-1.85986777702161e-09 7.82540023894543e-09 -1.8957321828871e-09;-1.7901190036642e-09 -1.8957321828871e-09 7.91264394645417e-09]  x1=[130.077722677422 9990.72598437802 9989.81518997748;314.159265358979 314.159265358979 314.159265358979;1.01767687081129 -0.17876493923835 -1.74971879982925]  x2=[130.078811942586 9990.55630473178 9989.64573670094;314.159265358979 314.159265358979 314.159265358979;1.01768277955904 -0.178772179827597 -1.7497259740102]  x3=[0.117310079985282 24.0456108626694 24.2381979628059;314.159265358979 314.159265358979 314.159265358979;0.998942413528294 -0.163438424554535 -1.73453038583969]  x4=[0.110176990039563 26.8001277837327 26.9932267966887;314.159265358979 314.159265358979 314.159265358979;1.0373662996277 -0.192715815885204 -1.76355684857313]  x5=8.14550361143895e-07  V1=ones(3,3)  V2=ones(3,3)  I1=ones(3,3)  I2=ones(3,3)  nHarmo=1  Measurements=None  Decoupling=off  VsMag0=0  VrMag0=0  VsAngle0=0  VrAngle0=0  IsMag0=0  IrMag0=0  IsAngle0=0  IrAngle0=0
      settings: SourceProductBaseCode=PS
  Line 72 : spsDistributedParametersLineLib/Distributed Parameters Line  Phases=3  Length=0.28  Frequency=50  Resistance=[0.646656091154803 0.0486237908083191 0.0486712220507153;0.0486237908083191 0.646561225344642 0.0486237934466192;0.0486712220507153 0.0486237934466192 0.646656091154803]  Inductance=[0.00282448912315926 0.00133270803418135 0.00132951476746136;0.00133270803418135 0.00282479813276775 0.00133799988507366;0.00132951476746136 0.00133799988507366 0.00282448912315926]  Capacitance=[7.89543174552926e-09 -1.85986777702161e-09 -1.7901190036642e-09;-1.85986777702161e-09 7.82540023894543e-09 -1.8957321828871e-09;-1.7901190036642e-09 -1.8957321828871e-09 7.91264394645417e-09]  x1=[130.064857368397 9993.10703347941 9992.19449396227;314.159265358979 314.159265358979 314.159265358979;1.01742230024893 -0.178813794167538 -1.7497688015237]  x2=[130.077722677422 9990.72598437802 9989.81518997748;314.159265358979 314.159265358979 314.159265358979;1.01751128940108 -0.178896482793706 -1.74985046860476]  x3=[0.144314051367367 14.7483960729621 14.9311579566324;314.159265358979 314.159265358979 314.159265358979;0.921696877088571 0.0856372642753648 -1.48809142919244]  x4=[0.0848893022496509 36.808268678046 37.0065053980257;314.159265358979 314.159265358979 314.159265358979;1.18018187727568 -0.284026100081259 -1.8546285412917]  x5=1.34161235953112e-06  V1=ones(3,3)  V2=ones(3,3)  I1=ones(3,3)  I2=ones(3,3)  nHarmo=1  Measurements=None  Decoupling=off  VsMag0=0  VrMag0=0  VsAngle0=0  VrAngle0=0  IsMag0=0  IrMag0=0  IsAngle0=0  IrAngle0=0
      settings: SourceProductBaseCode=PS
  Line 73 : spsDistributedParametersLineLib/Distributed Parameters Line  Phases=3  Length=0.01  Frequency=50  Resistance=[0.646656091154803 0.0486237908083191 0.0486712220507153;0.0486237908083191 0.646561225344642 0.0486237934466192;0.0486712220507153 0.0486237934466192 0.646656091154803]  Inductance=[0.00282448912315926 0.00133270803418135 0.00132951476746136;0.00133270803418135 0.00282479813276775 0.00133799988507366;0.00132951476746136 0.00133799988507366 0.00282448912315926]  Capacitance=[7.89543174552926e-09 -1.85986777702161e-09 -1.7901190036642e-09;-1.85986777702161e-09 7.82540023894543e-09 -1.8957321828871e-09;-1.7901190036642e-09 -1.8957321828871e-09 7.91264394645417e-09]  x1=[130.064397484775 9993.19205149176 9992.27944958032;314.159265358979 314.159265358979 314.159265358979;1.01782555025396 -0.178487959457168 -1.74944269590675]  x2=[130.064857368397 9993.10703347941 9992.19449396227;314.159265358979 314.159265358979 314.159265358979;1.01782872734672 -0.178490914531664 -1.74944561452927]  x3=[0.144331456923801 14.7540954799933 14.936959464457;314.159265358979 314.159265358979 314.159265358979;0.922092040823015 0.0858950665742598 -1.4878329295483]  x4=[0.0848966936708751 36.8233396251154 37.0217527674046;314.159265358979 314.159265358979 314.159265358979;1.18103977417622 -0.283391778361697 -1.85399374157336]  x5=4.79147271261115e-08  V1=ones(3,3)  V2=ones(3,3)  I1=ones(3,3)  I2=ones(3,3)  nHarmo=1  Measurements=None  Decoupling=off  VsMag0=0  VrMag0=0  VsAngle0=0  VrAngle0=0  IsMag0=0  IrMag0=0  IsAngle0=0  IrAngle0=0
      settings: SourceProductBaseCode=PS
  Line 74 : spsDistributedParametersLineLib/Distributed Parameters Line  Phases=3  Length=0.04  Frequency=50  Resistance=[0.646656091154803 0.0486237908083191 0.0486712220507153;0.0486237908083191 0.646561225344642 0.0486237934466192;0.0486712220507153 0.0486237934466192 0.646656091154803]  Inductance=[0.00282448912315926 0.00133270803418135 0.00132951476746136;0.00133270803418135 0.00282479813276775 0.00133799988507366;0.00132951476746136 0.00133799988507366 0.00282448912315926]  Capacitance=[7.89543174552926e-09 -1.85986777702161e-09 -1.7901190036642e-09;-1.85986777702161e-09 7.82540023894543e-09 -1.8957321828871e-09;-1.7901190036642e-09 -1.8957321828871e-09 7.91264394645417e-09]  x1=[130.062557668705 9993.53211012296 9992.6192585869;314.159265358979 314.159265358979 314.159265358979;1.01776768406889 -0.178512013357627 -1.74946692974412]  x2=[130.064397484775 9993.19205149176 9992.27944958032;314.159265358979 314.159265358979 314.159265358979;1.01778039168754 -0.178523834972265 -1.74947860557279]  x3=[0.144328692020342 14.7540746759891 14.9369332880405;314.159265358979 314.159265358979 314.159265358979;0.921988260506947 0.0857890869332745 -1.48793882061771]  x4=[0.0848951432490472 36.8223860961009 37.0207853903593;314.159265358979 314.159265358979 314.159265358979;1.18101214124091 -0.283417620700134 -1.85401961883804]  x5=1.91658908504446e-07  V1=ones(3,3)  V2=ones(3,3)  I1=ones(3,3)  I2=ones(3,3)  nHarmo=1  Measurements=None  Decoupling=off  VsMag0=0  VrMag0=0  VsAngle0=0  VrAngle0=0  IsMag0=0  IrMag0=0  IsAngle0=0  IrAngle0=0
      settings: SourceProductBaseCode=PS
  Line im3 : spsDistributedParametersLineLib/Distributed Parameters Line  Phases=3  Length=1e-10  Frequency=50  Resistance=[0.646656091154803 0.0486237908083191 0.0486712220507153;0.0486237908083191 0.646561225344642 0.0486237934466192;0.0486712220507153 0.0486237934466192 0.646656091154803]  Inductance=[0.00282448912315926 0.00133270803418135 0.00132951476746136;0.00133270803418135 0.00282479813276775 0.00133799988507366;0.00132951476746136 0.00133799988507366 0.00282448912315926]  Capacitance=[7.89543174552926e-09 -1.85986777702161e-09 -1.7901190036642e-09;-1.85986777702161e-09 7.82540023894543e-09 -1.8957321828871e-09;-1.7901190036642e-09 -1.8957321828871e-09 7.91264394645417e-09]  x1=[130.125187558175 9980.14784167968 9979.23767099227;314.159265358979 314.159265358979 314.159265358979;1.01840309761072 -0.178973580924593 -1.74992216038769]  x2=[130.125187558168 9980.14784167935 9979.23767099195;314.159265358979 314.159265358979 314.159265358979;1.01840309761066 -0.178973580924609 -1.74992216038771]  x3=[0.0783867541915792 20.7746120946321 21.1232664206954;314.159265358979 314.159265358979 314.159265358979;1.21705266158796 -0.126812314714434 -1.70118462629125]  x4=[0.161356421141279 30.0543339951648 30.0982845175431;314.159265358979 314.159265358979 314.159265358979;0.967902807848048 -0.215491354508124 -1.78382783848609]  x5=4.79147271261115e-16  V1=ones(3,3)  V2=ones(3,3)  I1=ones(3,3)  I2=ones(3,3)  nHarmo=1  Measurements=None  Decoupling=off  VsMag0=0  VrMag0=0  VsAngle0=0  VrAngle0=0  IsMag0=0  IrMag0=0  IsAngle0=0  IrAngle0=0
      settings: SourceProductBaseCode=PS
  Load 8041 : spsThreePhaseSeriesRLCLoadLib/Three-Phase Series RLC Load  LConnTagsString=A|B|C  Configuration=Delta  NominalVoltage=11000  Vabc=[1e3 1e3 1e3]  Vabcp=[1e3 1e3 1e3]  NominalFrequency=50  UnbalancedPower=off  ActivePower=28052.64  InductivePower=13586.514  CapacitivePower=0  Pabc=[10e3 9e3 11e3]  QLabc=[100 90 110]  QCabc=[100 90 110]  Pabcp=[10e3 9e3 11e3]  QLabcp=[100 90 110]  QCabcp=[100 90 110]  Measurements=None  LoadType=constant Z
  Load 8173 : spsThreePhaseSeriesRLCLoadLib/Three-Phase Series RLC Load  LConnTagsString=A|B|C  Configuration=Delta  NominalVoltage=11000  Vabc=[1e3 1e3 1e3]  Vabcp=[1e3 1e3 1e3]  NominalFrequency=50  UnbalancedPower=off  ActivePower=28052.64  InductivePower=13586.514  CapacitivePower=0  Pabc=[10e3 9e3 11e3]  QLabc=[100 90 110]  QCabc=[100 90 110]  Pabcp=[10e3 9e3 11e3]  QLabcp=[100 90 110]  QCabcp=[100 90 110]  Measurements=None  LoadType=constant Z
  Load 8287 : spsThreePhaseSeriesRLCLoadLib/Three-Phase Series RLC Load  LConnTagsString=A|B|C  Configuration=Delta  NominalVoltage=11000  Vabc=[1e3 1e3 1e3]  Vabcp=[1e3 1e3 1e3]  NominalFrequency=50  UnbalancedPower=off  ActivePower=35065.8  InductivePower=16983.142  CapacitivePower=0  Pabc=[10e3 9e3 11e3]  QLabc=[100 90 110]  QCabc=[100 90 110]  Pabcp=[10e3 9e3 11e3]  QLabcp=[100 90 110]  QCabcp=[100 90 110]  Measurements=None  LoadType=constant Z
  Load 8293 : spsThreePhaseSeriesRLCLoadLib/Three-Phase Series RLC Load  LConnTagsString=A|B|C  Configuration=Delta  NominalVoltage=11000  Vabc=[1e3 1e3 1e3]  Vabcp=[1e3 1e3 1e3]  NominalFrequency=50  UnbalancedPower=off  ActivePower=7013.16  InductivePower=3396.628  CapacitivePower=0  Pabc=[10e3 9e3 11e3]  QLabc=[100 90 110]  QCabc=[100 90 110]  Pabcp=[10e3 9e3 11e3]  QLabcp=[100 90 110]  QCabcp=[100 90 110]  Measurements=None  LoadType=constant Z
  Load 8424 : spsThreePhaseSeriesRLCLoadLib/Three-Phase Series RLC Load  LConnTagsString=A|B|C  Configuration=Delta  NominalVoltage=11000  Vabc=[1e3 1e3 1e3]  Vabcp=[1e3 1e3 1e3]  NominalFrequency=50  UnbalancedPower=off  ActivePower=11221.056  InductivePower=5434.605  CapacitivePower=0  Pabc=[10e3 9e3 11e3]  QLabc=[100 90 110]  QCabc=[100 90 110]  Pabcp=[10e3 9e3 11e3]  QLabcp=[100 90 110]  QCabcp=[100 90 110]  Measurements=None  LoadType=constant Z
  Load 8485 : spsThreePhaseSeriesRLCLoadLib/Three-Phase Series RLC Load  LConnTagsString=A|B|C  Configuration=Delta  NominalVoltage=11000  Vabc=[1e3 1e3 1e3]  Vabcp=[1e3 1e3 1e3]  NominalFrequency=50  UnbalancedPower=off  ActivePower=35065.8  InductivePower=16983.142  CapacitivePower=0  Pabc=[10e3 9e3 11e3]  QLabc=[100 90 110]  QCabc=[100 90 110]  Pabcp=[10e3 9e3 11e3]  QLabcp=[100 90 110]  QCabcp=[100 90 110]  Measurements=None  LoadType=constant Z
  Load 8551 : spsThreePhaseSeriesRLCLoadLib/Three-Phase Series RLC Load  LConnTagsString=A|B|C  Configuration=Delta  NominalVoltage=11000  Vabc=[1e3 1e3 1e3]  Vabcp=[1e3 1e3 1e3]  NominalFrequency=50  UnbalancedPower=off  ActivePower=11221.056  InductivePower=5434.605  CapacitivePower=0  Pabc=[10e3 9e3 11e3]  QLabc=[100 90 110]  QCabc=[100 90 110]  Pabcp=[10e3 9e3 11e3]  QLabcp=[100 90 110]  QCabcp=[100 90 110]  Measurements=None  LoadType=constant Z
  Load 8605 : spsThreePhaseSeriesRLCLoadLib/Three-Phase Series RLC Load  LConnTagsString=A|B|C  Configuration=Delta  NominalVoltage=11000  Vabc=[1e3 1e3 1e3]  Vabcp=[1e3 1e3 1e3]  NominalFrequency=50  UnbalancedPower=off  ActivePower=280.526  InductivePower=135.865  CapacitivePower=0  Pabc=[10e3 9e3 11e3]  QLabc=[100 90 110]  QCabc=[100 90 110]  Pabcp=[10e3 9e3 11e3]  QLabcp=[100 90 110]  QCabcp=[100 90 110]  Measurements=None  LoadType=constant Z
  Load 8733 : spsThreePhaseSeriesRLCLoadLib/Three-Phase Series RLC Load  LConnTagsString=A|B|C  Configuration=Delta  NominalVoltage=11000  Vabc=[1e3 1e3 1e3]  Vabcp=[1e3 1e3 1e3]  NominalFrequency=50  UnbalancedPower=off  ActivePower=7013.16  InductivePower=3396.628  CapacitivePower=0  Pabc=[10e3 9e3 11e3]  QLabc=[100 90 110]  QCabc=[100 90 110]  Pabcp=[10e3 9e3 11e3]  QLabcp=[100 90 110]  QCabcp=[100 90 110]  Measurements=None  LoadType=constant Z
  Load 8737 : spsThreePhaseSeriesRLCLoadLib/Three-Phase Series RLC Load  LConnTagsString=A|B|C  Configuration=Delta  NominalVoltage=11000  Vabc=[1e3 1e3 1e3]  Vabcp=[1e3 1e3 1e3]  NominalFrequency=50  UnbalancedPower=off  ActivePower=17532.9  InductivePower=8491.571  CapacitivePower=0  Pabc=[10e3 9e3 11e3]  QLabc=[100 90 110]  QCabc=[100 90 110]  Pabcp=[10e3 9e3 11e3]  QLabcp=[100 90 110]  QCabcp=[100 90 110]  Measurements=None  LoadType=constant Z
  R2 : spsThreePhaseVIMeasurementLib/Three-Phase V-I Measurement  VoltageMeasurement=phase-to-ground  SetLabelV=off  LabelV=Vabc  Vpu=off  VpuLL=off  CurrentMeasurement=yes  SetLabelI=off  LabelI=Iabc  Ipu=off  Pbase=100e6  Vbase=500e3  OutputType=Complex  PhasorSimulation=on  PSBequivalent=0
  R5 : spsThreePhaseVIMeasurementLib/Three-Phase V-I Measurement  VoltageMeasurement=phase-to-ground  SetLabelV=off  LabelV=Vabc  Vpu=off  VpuLL=off  CurrentMeasurement=yes  SetLabelI=off  LabelI=Iabc  Ipu=off  Pbase=100e6  Vbase=500e3  OutputType=Complex  PhasorSimulation=on  PSBequivalent=0
  Scope R2 : Scope  NumInputPorts=2
  Scope R5 : Scope  NumInputPorts=2
  Source PC1_TT2 : spsThreePhaseSourceLib/Three-Phase Source  InternalConnection=Yn  VoltagePhases=off  Voltage=10000  PhaseAngle=0  Voltage_phases=[25e3 25e3 25e3]/sqrt(3)  PhaseAngles_phases=[0 -120 +120]  Frequency=50  NonIdealSource=on  SpecifyImpedance=off  Resistance=0.14  Inductance=0.0031831  ShortCircuitLevel=100e6  BaseVoltage=25e3  XRratio=7  BusType=swing  Pref=10e3  Qref=0  Prefabc=[10e3, 10e3, 10e3]  Qrefabc=[0, 0, 0]  Qmin=-inf  Qmax=inf
  Source Zn : spsSeriesRLCBranchLib/Series RLC Branch  LConnTagsString=__new0  RConnTagsString=__new0  BranchType=RL  Resistance=0.001  Inductance=3.1831e-06  SetiL0=off  InitialCurrent=0  Capacitance=0  Setx0=off  InitialVoltage=0  Measurements=None
  powergui : spspowerguiLib/powergui  Priority=1  SimulationMode=Phasor  SampleTime=50e-6  frequency=50  Iterations=50  frequencyindice=50  Pbase=100e6  ErrMax=1e-4  UnitsV=kV  UnitsW=MW  buscounter=0  FunctionMessages=off  echomessages=off  EnableUseOfTLC=off  CurrentSourceSwitches=off  DisableSnubberDevices=off  DisableRonSwitches=off  DisableVfSwitches=off  DisplayEquations=off  AutomaticDiscreteSolvers=off  SolverType=Tustin/Backward Euler (TBE)  Interpol=off  ExternalGateDelay=off  methode=off  Ts=10  x0status=blocks  SPID=off  SwTol=0  HookPort=off  NonlinearTolerance=1e-4  nMaxIteration=100  ContinueOnMaxIteration=off  RestoreLinks=warning  ResistiveCurrentMeasurement=off  Frange=[0:2:500]  Ylog=off  Xlog=on  ShowGrid=off  save=off  variable=ZData  structure=0  ZoomFFT=off  StartTime=0.0  cycles=1  DisplayStyle=1  fundamental=60  FreqAxis=off  MaxFrequency=1000  frequencyindicesteady=1  RmsSteady=1  display=off
  wires:
  R2/1 -> Scope R2/1
  R2/2 -> Scope R2/2
  R5/1 -> Scope R5/1
  R5/2 -> Scope R5/2
  connections:
  Source Zn/LConn1 -- Ground/LConn1
  Source Zn/RConn1 -- Source PC1_TT2/LConn1
  Line 44/LConn1 -- Line 45/RConn1
  Line 44/LConn2 -- Line 45/RConn2
  Line 44/LConn3 -- Line 45/RConn3
  Line 47/LConn1 -- Line 46/RConn1
  Line 47/LConn2 -- Line 46/RConn2
  Line 47/LConn3 -- Line 46/RConn3
  Line 49/LConn1 -- Line 47/RConn1 -- Line 48/LConn1
  Line 49/LConn2 -- Line 47/RConn2 -- Line 48/LConn2
  Line 49/LConn3 -- Line 47/RConn3 -- Line 48/LConn3
  Line 50/LConn1 -- Line 51/RConn1
  Line 50/LConn2 -- Line 51/RConn2
  Line 50/LConn3 -- Line 51/RConn3
  Load 8737/LConn1 -- Line 52/RConn1
  Load 8737/LConn2 -- Line 52/RConn2
  Load 8737/LConn3 -- Line 52/RConn3
  Line 56/LConn1 -- Line 54/RConn1 -- Line 55/LConn1
  Line 56/LConn2 -- Line 54/RConn2 -- Line 55/LConn2
  Line 56/LConn3 -- Line 54/RConn3 -- Line 55/LConn3
  Line 58/LConn1 -- Line 56/RConn1 -- Line 57/LConn1
  Line 58/LConn2 -- Line 56/RConn2 -- Line 57/LConn2
  Line 58/LConn3 -- Line 56/RConn3 -- Line 57/LConn3
  Load 8293/LConn1 -- Line 57/RConn1
  Load 8293/LConn2 -- Line 57/RConn2
  Load 8293/LConn3 -- Line 57/RConn3
  Load 8551/LConn1 -- Line 58/RConn1
  Load 8551/LConn2 -- Line 58/RConn2
  Load 8551/LConn3 -- Line 58/RConn3
  Line 54/LConn1 -- Line 59/RConn1 -- Line 53/LConn1
  Line 54/LConn2 -- Line 59/RConn2 -- Line 53/LConn2
  Line 54/LConn3 -- Line 59/RConn3 -- Line 53/LConn3
  Line 61/LConn1 -- Line 60/RConn1
  Line 61/LConn2 -- Line 60/RConn2
  Line 61/LConn3 -- Line 60/RConn3
  R5/LConn1 -- Line 62/RConn1
  R5/LConn2 -- Line 62/RConn2
  R5/LConn3 -- Line 62/RConn3
  Load 8733/LConn1 -- Line 63/RConn1
  Load 8733/LConn2 -- Line 63/RConn2
  Load 8733/LConn3 -- Line 63/RConn3
  Line 63/LConn1 -- Line 64/RConn1 -- Line 62/LConn1
  Line 63/LConn2 -- Line 64/RConn2 -- Line 62/LConn2
  Line 63/LConn3 -- Line 64/RConn3 -- Line 62/LConn3
  Load 8485/LConn1 -- Line 65/RConn1 -- Line 64/LConn1
  Load 8485/LConn2 -- Line 65/RConn2 -- Line 64/LConn2
  Load 8485/LConn3 -- Line 65/RConn3 -- Line 64/LConn3
  Load 8605/LConn1 -- Line 66/RConn1
  Load 8605/LConn2 -- Line 66/RConn2
  Load 8605/LConn3 -- Line 66/RConn3
  Line 66/LConn1 -- Line 67/RConn1 -- Line 65/LConn1
  Line 66/LConn2 -- Line 67/RConn2 -- Line 65/LConn2
  Line 66/LConn3 -- Line 67/RConn3 -- Line 65/LConn3
  Line 69/LConn1 -- Line 68/RConn1
  Line 69/LConn2 -- Line 68/RConn2
  Line 69/LConn3 -- Line 68/RConn3
  Load 8287/LConn1 -- Line 69/RConn1
  Load 8287/LConn2 -- Line 69/RConn2
  Load 8287/LConn3 -- Line 69/RConn3
  Line 68/LConn1 -- Line 70/RConn1 -- Line 67/LConn1
  Line 68/LConn2 -- Line 70/RConn2 -- Line 67/LConn2
  Line 68/LConn3 -- Line 70/RConn3 -- Line 67/LConn3
  Load 8041/LConn1 -- Line 71/RConn1
  Load 8041/LConn2 -- Line 71/RConn2
  Load 8041/LConn3 -- Line 71/RConn3
  Line 71/LConn1 -- Line 72/RConn1 -- Line 70/LConn1
  Line 71/LConn2 -- Line 72/RConn2 -- Line 70/LConn2
  Line 71/LConn3 -- Line 72/RConn3 -- Line 70/LConn3
  Line 72/LConn1 -- Line 73/RConn1
  Line 72/LConn2 -- Line 73/RConn2
  Line 72/LConn3 -- Line 73/RConn3
  Line 73/LConn1 -- Line 74/RConn1
  Line 73/LConn2 -- Line 74/RConn2
  Line 73/LConn3 -- Line 74/RConn3
  Line 60/LConn1 -- Line im3/RConn1 -- Line 59/LConn1
  Line 60/LConn2 -- Line im3/RConn2 -- Line 59/LConn2
  Line 60/LConn3 -- Line im3/RConn3 -- Line 59/LConn3
  Line 74/LConn1 -- R2/RConn1
  Line 74/LConn2 -- R2/RConn2
  Line 74/LConn3 -- R2/RConn3
  Line im3/LConn1 -- R5/RConn1
  Line im3/LConn2 -- R5/RConn2
  Line im3/LConn3 -- R5/RConn3
  Source PC1_TT2/RConn1 -- R2/LConn1
  Source PC1_TT2/RConn2 -- R2/LConn2
  Source PC1_TT2/RConn3 -- R2/LConn3
  Line 51/LConn1 -- Line 52/LConn1 -- Line 53/RConn1
  Line 51/LConn2 -- Line 52/LConn2 -- Line 53/RConn2
  Line 51/LConn3 -- Line 52/LConn3 -- Line 53/RConn3
  Line 46/LConn1 -- Load 8173/LConn1 -- Line 50/RConn1 -- Line 45/LConn1
  Line 46/LConn2 -- Load 8173/LConn2 -- Line 50/RConn2 -- Line 45/LConn2
  Line 46/LConn3 -- Load 8173/LConn3 -- Line 50/RConn3 -- Line 45/LConn3
  Line 55/RConn1 -- Load 8424/LConn1
  Line 55/RConn2 -- Load 8424/LConn2
  Line 55/RConn3 -- Load 8424/LConn3
